simulink model "CarrotPlannerAlgorithm"  (R2022a)
settings: Solver=ode23s  StartTime=0.0  StopTime=inf  FixedStep=0.005  RelTol=1e-3
InitFcn:
  | RPInit
model workspace (MAT data in the model file):
  mapForSim : object (value not decoded)
  occGrid : robotics.BinaryOccupancyGrid (value not decoded)
undefined symbols (not defined in the file or in its folder): FloorSurface, Ref, RobotSurface, X, Y, Z
libraries: sm_lib x21, RoboticsPlayground x20, RP_Simulator_Components x15, nesl_utility x14
(part 2 of 2)

== stateflow chart CarrotPlannerAlgorithm/Vortex ==
  state TurningWest5
    LeftMotor=110;
    RightMotor=127;
  state TurningWest6
    LeftMotor=127;
    RightMotor=126;
  state TurningWest4
    LeftMotor=80;
    RightMotor=127;
  state TurningWest3
    LeftMotor=70;
    RightMotor=127;
  state rightFast8
    LeftMotor=125;
    RightMotor=127;
  state TurningWest
    LeftMotor=-40;
    RightMotor=80;
  state TurningWest2
    LeftMotor=40;
    RightMotor=127;
  state rightFast7
    LeftMotor=125;
    RightMotor=127;
  state StartingParameter
    LeftMotor=+127;
    RightMotor=+127;
  state TurningNorth
    LeftMotor=-40;
    RightMotor=80;
  state TurningNorth2
    LeftMotor=40;
    RightMotor=127;
  state TurningNorth3
    LeftMotor=70;
    RightMotor=127;
  state TurningNorth4
    LeftMotor=80;
    RightMotor=127;
  state TurningNorth5
    LeftMotor=110;
    RightMotor=127;
  state TurningNorth6
    LeftMotor=127;
    RightMotor=126;
  state TurningSouth6
    LeftMotor=126;
    RightMotor=127;
  state TurningSouth
    LeftMotor=-40;
    RightMotor=80;
  state TurningSouth2
    LeftMotor=40;
    RightMotor=127;
  state TurningSouth3
    LeftMotor=70;
    RightMotor=127;
  state TurningSouth4
    LeftMotor=80;
    RightMotor=127;
  state TurningSouth5
    LeftMotor=110;
    RightMotor=127;
  state rightFast10
    LeftMotor=127;
    RightMotor=125;
  state TurningSouth7
    LeftMotor=126;
    RightMotor=127;
  state TurningSouth11
    LeftMotor=80;
    RightMotor=-40;
  state TurningSouth12
    LeftMotor=127;
    RightMotor=40;
  state TurningSouth10
    LeftMotor=127;
    RightMotor=70;
  state TurningSouth9
    LeftMotor=127;
    RightMotor=80;
  state TurningSouth8
    LeftMotor=127;
    RightMotor=110;
  state rightFast9
    LeftMotor=127;
    RightMotor=125;
  state TurningSouth15
    LeftMotor=126;
    RightMotor=127;
  state TurningSouth16
    LeftMotor=-40;
    RightMotor=80;
  state TurningSouth17
    LeftMotor=40;
    RightMotor=127;
  state TurningSouth13
    LeftMotor=70;
    RightMotor=127;
  state TurningSouth18
    LeftMotor=80;
    RightMotor=127;
  state TurningSouth14
    LeftMotor=110;
    RightMotor=127;
  state TurningNorth9
    LeftMotor=-40;
    RightMotor=80;
  state TurningNorth12
    LeftMotor=40;
    RightMotor=127;
  state TurningNorth10
    LeftMotor=70;
    RightMotor=127;
  state TurningNorth11
    LeftMotor=80;
    RightMotor=127;
  state TurningNorth8
    LeftMotor=110;
    RightMotor=127;
  state TurningNorth7
    LeftMotor=126;
    RightMotor=127;
  state rightFast11
    LeftMotor=127;
    RightMotor=125;
  state TurningNorth15
    LeftMotor=0;
    RightMotor=0;
  rightFast7 -> StartingParameter [order 1] : [frontDist<0.3+(k*j)]{i=i+1;}
  rightFast8 -> StartingParameter [order 1] : [frontDist<0.3+(k*j)]{i=i+1;}
  rightFast8 -> TurningWest6 [order 2] : [180-angle>=0]
  TurningWest5 -> TurningWest6 : [180-angle>=0.1]
  TurningWest4 -> TurningWest5 : [180-angle<0.5]
  TurningWest3 -> TurningWest4 : [180-angle<2]
  StartingParameter -> TurningWest [order 2] : [frontDist<0.4+(k*j) && mod(i,3)==1 && rightDist<0.4+(k*j) && ~(j==4)]
  TurningWest2 -> TurningWest3 : [180-angle<5]
  TurningWest6 -> rightFast8 : [180-angle<0.1  || frontDist<0.3+(k*j)]
  TurningWest -> TurningWest2 : [180-angle<10]
  rightFast7 -> TurningNorth6 [order 2] : [180-angle<89.9]
  StartingParameter -> TurningNorth [order 1] : [frontDist<0.3+((k*j)-l*0.1) && mod(i,3)==0 && rightDist<0.3+(k*j) && ~(j==4)]
  TurningNorth -> TurningNorth2 : [180-angle<100]
  TurningNorth2 -> TurningNorth3 : [180-angle<95]
  TurningNorth3 -> TurningNorth4 : [180-angle<92]
  TurningNorth4 -> TurningNorth5 : [(180-angle<90.5)]
  TurningNorth5 -> TurningNorth6 : [180-angle<=(90.1)]
  (default) -> StartingParameter : {i=0, j=0,k=0.3,l=0}
  TurningNorth6 -> rightFast7 : [180-angle>=90 || frontDist<0.3+(k*j)]
  StartingParameter -> TurningNorth15 [order 3] : [j==4 && leftDist<0.1]
  rightFast11 -> StartingParameter [order 2] : [frontDist<0.3+(k*j)]{i=0;}
  TurningSouth6 -> StartingParameter : {i=i+1;}
  StartingParameter -> TurningSouth11 [order 4] : [mod(i,3)==0 && rightDist>=0.3+(k*j) && frontDist<4-(k*j) && ~(j==4)]
  StartingParameter -> TurningSouth [order 5] : [frontDist<0.3+((k*j)-l*0.1) && mod(i,3)==2 && rightDist<0.3+(k*j) && ~(j==4)]
  TurningSouth -> TurningSouth2 : [angle<100]
  TurningSouth2 -> TurningSouth3 : [angle<95]
  TurningSouth3 -> TurningSouth4 : [angle<92]
  TurningSouth4 -> TurningSouth5 : [angle<90.5]
  TurningSouth5 -> TurningSouth6 : [angle<=(90.1)]
  rightFast10 -> TurningSouth15 : [angle>90 || frontDist<0.3+(k*j)]
  TurningSouth15 -> rightFast10 [order 1] : [angle<=90.1 && ~(frontDist<0.3+(k*j))]
  TurningSouth11 -> TurningSouth12 : [180-angle<10]
  TurningSouth12 -> TurningSouth10 : [180-angle<5]
  TurningSouth10 -> TurningSouth9 : [180-angle<2]
  TurningSouth9 -> TurningSouth8 : [180-angle<0.5]
  TurningSouth8 -> TurningSouth7 : [180-angle<=0.1]
  TurningSouth7 -> rightFast9 : [180-angle>=0.1  || frontDist<0.3+(k*j)]
  rightFast9 -> TurningSouth7 [order 1] : [180-angle<0.1]
  rightFast9 -> TurningSouth16 [order 2] : [frontDist<0.3+(k*j) && rightDist<0.3+(k*j) && ~(j==4) ]{j=j+1;l=l+1}
  TurningSouth16 -> TurningSouth17 : [angle<100]
  TurningSouth17 -> TurningSouth13 : [angle<95]
  TurningSouth13 -> TurningSouth18 : [angle<92]
  TurningSouth18 -> TurningSouth14 : [angle<90.5]
  TurningSouth14 -> TurningSouth15 : [angle<=(90.1)]
  TurningNorth9 -> TurningNorth12 : [angle<10]
  TurningNorth12 -> TurningNorth10 : [angle<5]
  TurningNorth10 -> TurningNorth11 : [angle<2]
  TurningNorth11 -> TurningNorth8 : [(angle<0.5)]
  TurningNorth8 -> TurningNorth7 : [angle<=0.1]
  TurningSouth15 -> TurningNorth9 [order 2] : [frontDist<0.3+(k*j) && rightDist<0.3+(k*j)]
  TurningNorth7 -> rightFast11 : [angle>=0.1  || frontDist<0.3+(k*j)]
  rightFast11 -> TurningNorth7 [order 1] : [angle<0.1 && ~(frontDist<0.3+(k*j))]
  data: LeftMotor output; RightMotor output; frontDist input; leftDist input; rightDist input; angle input; i local; xpose input; ypose input; j local; k local; dir input; l local

== stateflow chart CarrotPlannerAlgorithm/S pattern1 ==
  state rightFast7
    LeftMotor=125;
    RightMotor=127;
  state ControlPart5
    LeftMotor=127;
    RightMotor=125;
  state rightFast6
    LeftMotor=127;
    RightMotor=126;
  state rightFast5
    LeftMotor=127;
    RightMotor=110;
  state leftFast5
    LeftMotor=110;
    RightMotor=127;
  state ControlPart6
    LeftMotor=126;
    RightMotor=127;
  state rightFast4
    LeftMotor=127;
    RightMotor=80;
  state leftFast4
    LeftMotor=80;
    RightMotor=127;
  state Initial1
    LeftMotor=127;
    RightMotor=+127;
  state rightFast1
    LeftMotor=80;
    RightMotor=-40;
  state rightFast2
    LeftMotor=127;
    RightMotor=40;
  state rightFast3
    LeftMotor=127;
    RightMotor=70;
  state leftFast1
    LeftMotor=-40;
    RightMotor=80;
  state leftFast3
    LeftMotor=70;
    RightMotor=127;
  state leftFast2
    LeftMotor=40;
    RightMotor=127;
  state Init1
    LeftMotor=-80;
    RightMotor=80;;
  state Init2
    LeftMotor=-50;
    RightMotor=50;
  state StartCond
    x = abs(xpose-xdesired);
    y = abs(ypose-ydesired);
    alfa = atan(y/x);
    alfa = rad2deg(alfa);
    alfa1=alfa;
    out=0;
  state Init3
    LeftMotor=-30;
    RightMotor=30;
  state Init7
    LeftMotor=123;
    RightMotor=120;
  state Init5
    LeftMotor=100;
    RightMotor=100;
  state Init6
    LeftMotor=120;
    RightMotor=121.3;
  state Init17
    out=0;
    LeftMotor=-80;
    RightMotor=80;
  state rightFast10
    LeftMotor=125;
    RightMotor=127;
  state abcd2
    LeftMotor=-50;
    RightMotor=50;
  state ControlPart8
    LeftMotor=127;
    RightMotor=125;
  state rightFast8
    LeftMotor=127;
    RightMotor=126;
  state rightFast11
    LeftMotor=127;
    RightMotor=110;
  state abcd
    LeftMotor=-30;
    RightMotor=30;
  state leftFast9
    LeftMotor=110;
    RightMotor=127;
  state ControlPart7
    LeftMotor=126;
    RightMotor=127;
  state abcd1
    LeftMotor=-10;
    RightMotor=10;
  state rightFast9
    LeftMotor=127;
    RightMotor=80;
  state leftFast10
    LeftMotor=80;
    RightMotor=127;
  state abcd3
    LeftMotor=3;
    RightMotor=-3;
  state Initial2
    LeftMotor=127;
    RightMotor=127;
  state rightFast14
    LeftMotor=80;
    RightMotor=-40;
  state rightFast12
    LeftMotor=127;
    RightMotor=40;
  state rightFast13
    LeftMotor=127;
    RightMotor=70;
  state leftFast6
    LeftMotor=-40;
    RightMotor=80;
  state leftFast7
    LeftMotor=70;
    RightMotor=127;
  state leftFast8
    LeftMotor=40;
    RightMotor=127;
  rightFast7 -> rightFast6 : [angle<0.1 || frontDist<0.3]
  rightFast6 -> rightFast7 [order 1] : [angle>=0.1 && ~(frontDist<0.3)]
  ControlPart5 -> ControlPart6 : [angle>179.9 || frontDist<0.3]
  ControlPart6 -> ControlPart5 [order 1] : [dir==0 &&angle>=0.1 && ~(frontDist<0.3)]
  rightFast6 -> Initial1 [order 2] : [(frontDist<0.3 &&mod(i,2)==0)]
  rightFast5 -> rightFast6 : [angle<(0.2)]{i=i+1;}
  rightFast4 -> rightFast5 : [angle>0&&angle<0.5]
  leftFast5 -> ControlPart6 : [180-angle<(0.2)]{i=i+1;}
  leftFast4 -> leftFast5 : [180-angle<0.5]
  ControlPart6 -> Initial1 [order 2] : [frontDist<0.3 &&mod(i,2)==1]
  (default) -> Initial1 : {i=0,j=0,k=0}
  rightFast3 -> rightFast4 : [angle>0&&angle<2]
  leftFast3 -> leftFast4 : [180-angle<2]
  Initial1 -> rightFast1 [order 1] : [frontDist<0.3 &&mod(i,2)==1 && ~(i==17)]
  Initial1 -> leftFast1 [order 3] : [frontDist<0.3 &&mod(i,2)==0 && ~(i==17)]
  rightFast1 -> rightFast2 : [angle>0&&angle<10]
  rightFast2 -> rightFast3 : [angle>0&&angle<5]
  leftFast1 -> leftFast2 : [180-angle<10]
  leftFast2 -> leftFast3 : [180-angle<5]
  Initial1 -> StartCond [order 2] : [i==17]{xdesired=4.8;ydesired=3;}
  StartCond -> Init1
  Init1 -> Init2 : [abs(angle-alfa)<3]
  Init2 -> Init3 : [abs(angle-alfa)<1]
  Init3 -> Init5 : [abs(angle-alfa)<0.2]
  Init5 -> Init7 [order 3] : [[angle-alfa<0.5]]
  Init6 -> Init5 [order 2] : [alfa-angle<0.005]
  Init7 -> Init5 [order 2] : [[[angle-alfa<0.1]]]
  Init5 -> Init6 [order 2] : [alfa-angle<0.1]
  Init7 -> Init17 [order 1] : [xdesired-xpose<0.005 && ydesired-ypose<0.005 ]
  Init5 -> Init17 [order 1] : [xdesired-xpose<0.005 && ydesired-ypose<0.005 ]
  Init6 -> Init17 [order 1] : [xdesired-xpose<0.005 && ydesired-ypose<0.005 ]
  Init17 -> abcd2 : [angle<10]
  rightFast10 -> rightFast8 : [angle<179.9 || frontDist<0.3]
  rightFast8 -> rightFast10 [order 1] : [angle>=180 && ~(frontDist<0.3)]
  abcd2 -> abcd : [angle<2]
  ControlPart8 -> ControlPart7 : [angle>0.1 || frontDist<0.3]
  ControlPart7 -> ControlPart8 [order 1] : [dir==0 &&angle<=0 && ~(frontDist<0.3)]
  rightFast8 -> Initial2 [order 2] : [(frontDist<0.3 &&mod(i,2)==0)]
  rightFast11 -> rightFast8 : [angle>179.8 && angle<180]{i=i+1;}
  abcd -> abcd1 : [angle<0.5]
  rightFast9 -> rightFast11 : [angle>179.5 && angle<180]
  leftFast9 -> ControlPart7 : [angle<(0.2)]{i=i+1;}
  leftFast10 -> leftFast9 : [angle<0.5]
  ControlPart7 -> Initial2 [order 2] : [frontDist<0.3 &&mod(i,2)==1]
  abcd1 -> abcd3 : [angle<0.2]
  rightFast13 -> rightFast9 : [angle>178 && angle<180]
  leftFast7 -> leftFast10 : [angle<2]
  abcd3 -> Initial2 : [0.1>angle]
  Initial2 -> rightFast14 [order 1] : [frontDist<0.3 &&mod(i,2)==1]
  Initial2 -> leftFast6 [order 2] : [frontDist<0.3 &&mod(i,2)==0]
  rightFast14 -> rightFast12 : [angle>170 && angle<180]
  rightFast12 -> rightFast13 : [angle>175 && angle<180]
  leftFast6 -> leftFast8 : [angle<10]
  leftFast8 -> leftFast7 : [angle<5]
  data: LeftMotor output; RightMotor output; frontDist input; leftDist input; rightDist input; angle input; i local; xpose input; ypose input; j local; k local; dir input; alfa1 output; out output; xdesired local; x local; ydesired local; y local; alfa local

== stateflow chart CarrotPlannerAlgorithm/Vortex3 ==
  state TurningWest5
    LeftMotor=110;
    RightMotor=127;
  state TurningWest6
    LeftMotor=127;
    RightMotor=126;
  state TurningWest4
    LeftMotor=80;
    RightMotor=127;
  state TurningWest3
    LeftMotor=70;
    RightMotor=127;
  state rightFast8
    LeftMotor=125;
    RightMotor=127;
  state TurningWest
    LeftMotor=-40;
    RightMotor=80;
  state TurningWest2
    LeftMotor=40;
    RightMotor=127;
  state rightFast7
    LeftMotor=125;
    RightMotor=127;
  state StartingParameter
    LeftMotor=+127;
    RightMotor=+127;
  state TurningNorth
    LeftMotor=-40;
    RightMotor=80;
  state TurningNorth2
    LeftMotor=40;
    RightMotor=127;
  state TurningNorth3
    LeftMotor=70;
    RightMotor=127;
  state TurningNorth4
    LeftMotor=80;
    RightMotor=127;
  state TurningNorth5
    LeftMotor=110;
    RightMotor=127;
  state TurningNorth6
    LeftMotor=127;
    RightMotor=126;
  state TurningSouth6
    LeftMotor=126;
    RightMotor=127;
  state TurningSouth
    LeftMotor=-40;
    RightMotor=80;
  state TurningSouth2
    LeftMotor=40;
    RightMotor=127;
  state TurningSouth3
    LeftMotor=70;
    RightMotor=127;
  state TurningSouth4
    LeftMotor=80;
    RightMotor=127;
  state TurningSouth5
    LeftMotor=110;
    RightMotor=127;
  state TurningSouth7
    LeftMotor=126;
    RightMotor=127;
  state TurningSouth11
    LeftMotor=80;
    RightMotor=-40;
  state TurningSouth12
    LeftMotor=127;
    RightMotor=40;
  state TurningSouth10
    LeftMotor=127;
    RightMotor=70;
  state TurningSouth9
    LeftMotor=127;
    RightMotor=80;
  state TurningSouth8
    LeftMotor=127;
    RightMotor=110;
  state StartCond
    x = abs(xpose-xdesired);
    y = abs(ypose-ydesired);
    alfa = atan(y/x);
    alfa = rad2deg(alfa);
    alfa1=alfa;
    out=0;
  state TurningWest15
    LeftMotor=127;
    RightMotor=126;
  state TurningWest7
    LeftMotor=127;
    RightMotor=126;
  state Init1
    LeftMotor=80;
    RightMotor=-80;;
  state Init2
    LeftMotor=50;
    RightMotor=-50;
  state TurningSouth23
    LeftMotor=-40;
    RightMotor=80;
  state TurningNorth23
    LeftMotor=126;
    RightMotor=127;
  state TurningNorth27
    LeftMotor=-40;
    RightMotor=80;
  state rightFast11
    LeftMotor=127;
    RightMotor=125;
  state TurningNorth18
    LeftMotor=-40;
    RightMotor=80;
  state rightFast9
    LeftMotor=127;
    RightMotor=125;
  state TurningNorth7
    LeftMotor=126;
    RightMotor=127;
  state TurningSouth16
    LeftMotor=-40;
    RightMotor=80;
  state Init4
    LeftMotor=10;
    RightMotor=-10;
  state Init3
    LeftMotor=30;
    RightMotor=-30;
  state TurningWest18
    LeftMotor=110;
    RightMotor=127;
  state TurningNorth20
    LeftMotor=110;
    RightMotor=127;
  state TurningNorth8
    LeftMotor=110;
    RightMotor=127;
  state TurningSouth17
    LeftMotor=40;
    RightMotor=127;
  state TurningWest9
    LeftMotor=110;
    RightMotor=127;
  state TurningSouth24
    LeftMotor=40;
    RightMotor=127;
  state TurningNorth29
    LeftMotor=40;
    RightMotor=127;
  state TurningNorth16
    LeftMotor=40;
    RightMotor=127;
  state TurningSouth13
    LeftMotor=70;
    RightMotor=127;
  state TurningNorth11
    LeftMotor=80;
    RightMotor=127;
  state Init7
    LeftMotor=120;
    RightMotor=123;
  state Init5
    LeftMotor=100;
    RightMotor=100;
  state Init6
    LeftMotor=121.3;
    RightMotor=120;
  state TurningNorth28
    LeftMotor=70;
    RightMotor=127;
  state TurningNorth14
    LeftMotor=70;
    RightMotor=127;
  state TurningSouth21
    LeftMotor=70;
    RightMotor=127;
  state TurningNorth19
    LeftMotor=80;
    RightMotor=127;
  state TurningWest13
    LeftMotor=80;
    RightMotor=127;
  state TurningWest11
    LeftMotor=80;
    RightMotor=127;
  state TurningSouth18
    LeftMotor=80;
    RightMotor=127;
  state TurningNorth10
    LeftMotor=70;
    RightMotor=127;
  state TurningWest16
    LeftMotor=70;
    RightMotor=127;
  state TurningNorth25
    LeftMotor=80;
    RightMotor=127;
  state TurningWest10
    LeftMotor=70;
    RightMotor=127;
  state TurningSouth19
    LeftMotor=80;
    RightMotor=127;
  state TurningNorth13
    LeftMotor=80;
    RightMotor=127;
  state TurningNorth21
    LeftMotor=70;
    RightMotor=127;
  state Init17
    out=0;
    LeftMotor=80;
    RightMotor=-80;
  state TurningSouth14
    LeftMotor=110;
    RightMotor=127;
  state TurningNorth12
    LeftMotor=40;
    RightMotor=127;
  state TurningWest17
    LeftMotor=40;
    RightMotor=127;
  state TurningNorth30
    LeftMotor=110;
    RightMotor=127;
  state TurningWest12
    LeftMotor=40;
    RightMotor=127;
  state TurningNorth15
    LeftMotor=110;
    RightMotor=127;
  state TurningSouth20
    LeftMotor=110;
    RightMotor=127;
  state TurningNorth22
    LeftMotor=40;
    RightMotor=127;
  state abcd2
    LeftMotor=50;
    RightMotor=-50;
  state TurningSouth15
    LeftMotor=126;
    RightMotor=127;
  state rightFast10
    LeftMotor=127;
    RightMotor=125;
  state TurningNorth9
    LeftMotor=-40;
    RightMotor=80;
  state TurningWest14
    LeftMotor=-40;
    RightMotor=80;
  state TurningNorth26
    LeftMotor=127;
    RightMotor=126;
  state TurningWest8
    LeftMotor=-40;
    RightMotor=80;
  state TurningSouth22
    LeftMotor=126;
    RightMotor=127;
  state TurningNorth17
    LeftMotor=127;
    RightMotor=126;
  state TurningNorth24
    LeftMotor=-40;
    RightMotor=80;
  state abcd
    LeftMotor=30;
    RightMotor=-30;
  state abcd1
    LeftMotor=10;
    RightMotor=-10;
  state abcd3
    LeftMotor=3;
    RightMotor=-3;
  state Duz
    LeftMotor=126;
    RightMotor=127;
  state TurningWest21
    LeftMotor=127;
    RightMotor=126;
  state TurningSouth25
    LeftMotor=-40;
    RightMotor=80;
  state TurningNorth40
    LeftMotor=126;
    RightMotor=127;
  state TurningNorth33
    LeftMotor=-40;
    RightMotor=80;
  state TurningWest24
    LeftMotor=110;
    RightMotor=127;
  state TurningSouth28
    LeftMotor=40;
    RightMotor=127;
  state TurningNorth42
    LeftMotor=110;
    RightMotor=127;
  state TurningNorth35
    LeftMotor=40;
    RightMotor=127;
  state TurningSouth27
    LeftMotor=70;
    RightMotor=127;
  state TurningNorth38
    LeftMotor=80;
    RightMotor=127;
  state TurningWest19
    LeftMotor=80;
    RightMotor=127;
  state TurningNorth34
    LeftMotor=70;
    RightMotor=127;
  state TurningWest22
    LeftMotor=70;
    RightMotor=127;
  state TurningSouth29
    LeftMotor=80;
    RightMotor=127;
  state TurningNorth31
    LeftMotor=80;
    RightMotor=127;
  state TurningNorth41
    LeftMotor=70;
    RightMotor=127;
  state TurningWest23
    LeftMotor=40;
    RightMotor=127;
  state TurningNorth36
    LeftMotor=110;
    RightMotor=127;
  state TurningSouth30
    LeftMotor=110;
    RightMotor=127;
  state TurningNorth39
    LeftMotor=40;
    RightMotor=127;
  state TurningWest20
    LeftMotor=-40;
    RightMotor=80;
  state TurningSouth26
    LeftMotor=126;
    RightMotor=127;
  state TurningNorth32
    LeftMotor=127;
    RightMotor=126;
  state TurningNorth37
    LeftMotor=-40;
    RightMotor=80;
  rightFast7 -> StartingParameter [order 1] : [frontDist<0.3+(k*j)]{i=i+1;}
  rightFast8 -> StartingParameter [order 1] : [frontDist<0.3+(k*j)]{i=i+1;}
  rightFast8 -> TurningWest6 [order 2] : [180-angle>=0]
  TurningWest5 -> TurningWest6 : [180-angle>=0.1]
  TurningWest4 -> TurningWest5 : [180-angle<0.5]
  TurningWest3 -> TurningWest4 : [180-angle<2]
  StartingParameter -> TurningWest [order 2] : [frontDist<0.3+(k*j) && mod(i,3)==1 && rightDist<0.3+(k*j) || leftDist<0.3]
  TurningWest2 -> TurningWest3 : [180-angle<5]
  TurningWest6 -> rightFast8 : [180-angle<0.1  || frontDist<0.3+(k*j)]
  TurningWest -> TurningWest2 : [180-angle<10]
  rightFast7 -> TurningNorth6 [order 2] : [180-angle<89.9]
  StartingParameter -> TurningNorth [order 1] : [frontDist<0.2+((k*j)) && mod(i,3)==0 && rightDist<0.3+(k*j)  || leftDist<0.3]
  TurningNorth -> TurningNorth2 : [180-angle<100]
  TurningNorth2 -> TurningNorth3 : [180-angle<95]
  TurningNorth3 -> TurningNorth4 : [180-angle<92]
  TurningNorth4 -> TurningNorth5 : [(180-angle<90.5)]
  TurningNorth5 -> TurningNorth6 : [180-angle<=(90.1)]
  (default) -> StartingParameter : {i=0, j=0,k=0.3,l=0}
  TurningNorth6 -> rightFast7 : [180-angle>=90 || frontDist<0.3+(k*j)]
  rightFast11 -> StartingParameter [order 3] : [frontDist<0.3+(k*j)]{i=0;}
  TurningSouth6 -> StartingParameter : {i=i+1;}
  StartingParameter -> TurningSouth11 [order 3] : [mod(i,3)==0 && rightDist>=0.3+(k*j) && frontDist<4-(k*j)  || leftDist<0.3]
  StartingParameter -> TurningSouth [order 4] : [frontDist<0.3+((k*j)) && mod(i,3)==2 && rightDist<0.3+(k*j)  || leftDist<0.3]
  TurningSouth -> TurningSouth2 : [angle<100]
  TurningSouth2 -> TurningSouth3 : [angle<95]
  TurningSouth3 -> TurningSouth4 : [angle<92]
  TurningSouth4 -> TurningSouth5 : [angle<90.5]
  TurningSouth5 -> TurningSouth6 : [angle<=(90.1)]
  TurningSouth11 -> TurningSouth12 : [180-angle<10]
  TurningSouth12 -> TurningSouth10 : [180-angle<5]
  TurningSouth10 -> TurningSouth9 : [180-angle<2]
  TurningSouth9 -> TurningSouth8 : [180-angle<0.5]
  TurningSouth8 -> TurningSouth7 : [180-angle<=0.1]
  TurningSouth7 -> rightFast9 : [180-angle>=0.1  || frontDist<0.3+(k*j)]
  rightFast9 -> TurningSouth7 [order 1] : [180-angle<0.1]
  TurningWest15 -> StartCond : [frontDist<=1.7]{xdesired=3;ydesired=3.6;}
  StartCond -> Init1
  Init1 -> Init2 : [abs(angle-alfa)<5]
  TurningWest7 -> TurningSouth23 : [frontDist<1.5]
  TurningNorth23 -> TurningNorth27 : [frontDist<0.8]
  rightFast11 -> TurningNorth18 [order 2] : [frontDist<=3 && l==8]
  rightFast11 -> TurningNorth7 [order 1] : [angle<0.1 && ~(frontDist<0.3+(k*j))]
  rightFast9 -> TurningSouth16 [order 2] : [frontDist<0.3+(k*j) && rightDist<0.3+(k*j) || leftDist<0.3]{j=j+1;l=l+1}
  Init2 -> Init3 : [abs(angle-alfa)<3]
  TurningSouth23 -> TurningSouth24 : [angle<100]
  TurningNorth20 -> TurningNorth23 : [angle<=0.1]
  TurningNorth27 -> TurningNorth29 : [180-angle<100]
  TurningWest18 -> TurningWest15 : [180-angle>=0.1]
  TurningNorth7 -> rightFast11 : [angle>=0.1  || frontDist<0.3+(k*j)]
  TurningWest9 -> TurningWest7 : [180-angle>=0.1]
  TurningNorth18 -> TurningNorth16 : [180-angle<100]
  TurningNorth8 -> TurningNorth7 : [angle<=0.1]
  TurningSouth16 -> TurningSouth17 : [angle<100]
  Init3 -> Init4 : [abs(angle-alfa)<1]
  Init4 -> Init5 : [abs(angle-alfa)<0.3]
  TurningNorth19 -> TurningNorth20 : [(angle<0.5)]
  TurningNorth11 -> TurningNorth8 : [(angle<0.5)]
  TurningSouth17 -> TurningSouth13 : [angle<95]
  TurningSouth24 -> TurningSouth21 : [angle<95]
  TurningNorth29 -> TurningNorth28 : [180-angle<95]
  TurningWest13 -> TurningWest18 : [180-angle<0.5]
  TurningNorth16 -> TurningNorth14 : [180-angle<95]
  TurningWest11 -> TurningWest9 : [180-angle<0.5]
  Init5 -> Init7 [order 3] : [angle-alfa<0.5]
  Init6 -> Init5 [order 2] : [alfa-angle<0.005]
  Init7 -> Init5 [order 2] : [angle-alfa<0.1]
  Init5 -> Init6 [order 2] : [alfa-angle<0.1]
  TurningSouth13 -> TurningSouth18 : [angle<92]
  TurningNorth10 -> TurningNorth11 : [angle<2]
  Init7 -> Init17 [order 1] : [xdesired-xpose<0.005 && ydesired-ypose<0.005 ]
  Init6 -> Init17 [order 1] : [xdesired-xpose<0.005 && ydesired-ypose<0.005 ]
  Init5 -> Init17 [order 1] : [xdesired-xpose<0.005 && ydesired-ypose<0.005 ]
  TurningNorth28 -> TurningNorth25 : [180-angle<92]
  TurningNorth14 -> TurningNorth13 : [180-angle<92]
  TurningSouth21 -> TurningSouth19 : [angle<92]
  TurningNorth21 -> TurningNorth19 : [angle<2]
  TurningWest16 -> TurningWest13 : [180-angle<2]
  TurningWest10 -> TurningWest11 : [180-angle<2]
  TurningSouth18 -> TurningSouth14 : [angle<90.5]
  TurningNorth12 -> TurningNorth10 : [angle<5]
  TurningNorth25 -> TurningNorth30 : [(180-angle<90.5)]
  TurningWest17 -> TurningWest16 : [180-angle<5]
  TurningSouth19 -> TurningSouth20 : [angle<90.5]
  TurningNorth13 -> TurningNorth15 : [(180-angle<90.5)]
  TurningNorth22 -> TurningNorth21 : [angle<5]
  TurningWest12 -> TurningWest10 : [180-angle<5]
  Init17 -> abcd2 : [angle<10]
  TurningSouth14 -> TurningSouth15 : [angle<=(90.1)]{l=l+1;}
  TurningNorth9 -> TurningNorth12 : [angle<10]
  TurningNorth30 -> TurningNorth26 : [180-angle<=(90.1)]
  TurningWest14 -> TurningWest17 : [180-angle<10]
  TurningNorth15 -> TurningNorth17 : [180-angle<=(90.1)]
  TurningSouth20 -> TurningSouth22 : [angle<=(90.1)]
  TurningNorth24 -> TurningNorth22 : [angle<10]
  TurningWest8 -> TurningWest12 : [180-angle<10]
  TurningSouth15 -> rightFast10 [order 1] : [angle<=90.1 && ~(frontDist<0.3+(k*j))]
  abcd2 -> abcd : [angle<2]
  TurningSouth15 -> TurningNorth9 [order 2] : [frontDist<0.3+(k*j) && rightDist<0.3+(k*j)  || leftDist<0.3]
  rightFast10 -> TurningSouth15 : [angle>90 || frontDist<0.3+(k*j)]
  TurningNorth26 -> TurningWest14 : [frontDist<=3.6]
  TurningSouth22 -> TurningNorth24 : [frontDist<1.8]
  TurningNorth17 -> TurningWest8 : [frontDist<=3.2]
  abcd -> abcd1 : [angle<0.5]
  abcd1 -> abcd3 : [angle<0.2]
  abcd3 -> Duz : [0.1>=angle]
  Duz -> TurningNorth33 : [frontDist<=1.5]
  TurningWest21 -> TurningSouth25 : [frontDist<2.2]
  TurningSouth25 -> TurningNorth37 [order 2] : [frontDist<1.4]
  TurningSouth25 -> TurningSouth28 [order 1] : [angle<100]
  TurningNorth42 -> TurningNorth40 : [angle<=0.1]
  TurningWest24 -> TurningWest21 : [180-angle>=0.1]
  TurningNorth33 -> TurningNorth35 : [180-angle<100]
  TurningSouth28 -> TurningSouth27 : [angle<95]
  TurningNorth38 -> TurningNorth42 : [(angle<0.5)]
  TurningWest19 -> TurningWest24 : [180-angle<0.5]
  TurningNorth35 -> TurningNorth34 : [180-angle<95]
  TurningSouth27 -> TurningSouth29 : [angle<92]
  TurningNorth41 -> TurningNorth38 : [angle<2]
  TurningWest22 -> TurningWest19 : [180-angle<2]
  TurningNorth34 -> TurningNorth31 : [180-angle<92]
  TurningSouth29 -> TurningSouth30 : [angle<90.5]
  TurningNorth31 -> TurningNorth36 : [(180-angle<90.5)]
  TurningWest23 -> TurningWest22 : [180-angle<5]
  TurningNorth39 -> TurningNorth41 : [angle<5]
  TurningNorth36 -> TurningNorth32 : [180-angle<=(90.1)]
  TurningSouth30 -> TurningSouth26 : [angle<=(90.1)]
  TurningWest20 -> TurningWest23 : [180-angle<10]
  TurningNorth37 -> TurningNorth39 : [angle<10]
  TurningNorth32 -> TurningWest20 : [frontDist<1.4]
  data: LeftMotor output; RightMotor output; frontDist input; leftDist input; rightDist input; angle input; i local; xpose input; ypose input; j local; k local; dir input; l local; xdesired local; y local; alfa local; ydesired local; x local; alfa1 output; out output

== matlab function CarrotPlannerAlgorithm/MATLAB Function ==
  data: u input; y output
function y = fcn(u)
    if u<0
        y=0;
    else
        y=1;
    end

end

== stateflow chart CarrotPlannerAlgorithm/S pattern ==
  note: frontdistance'yi buraya ekleyip dene
  state rightFast7
    LeftMotor=125;
    RightMotor=127;
  state ControlPart5
    LeftMotor=127;
    RightMotor=125;
  state rightFast6
    LeftMotor=127;
    RightMotor=126;
  state rightFast5
    LeftMotor=127;
    RightMotor=110;
  state leftFast5
    LeftMotor=110;
    RightMotor=127;
  state ControlPart6
    LeftMotor=126;
    RightMotor=127;
  state rightFast4
    LeftMotor=127;
    RightMotor=80;
  state leftFast4
    LeftMotor=80;
    RightMotor=127;
  state Initial1
    LeftMotor=127;
    RightMotor=+127;
  state rightFast1
    LeftMotor=80;
    RightMotor=-40;
  state rightFast2
    LeftMotor=127;
    RightMotor=40;
  state rightFast3
    LeftMotor=127;
    RightMotor=70;
  state leftFast1
    LeftMotor=-40;
    RightMotor=80;
  state leftFast3
    LeftMotor=70;
    RightMotor=127;
  state leftFast2
    LeftMotor=40;
    RightMotor=127;
  state Stop
    LeftMotor=127;
    RightMotor=127;
  rightFast7 -> rightFast6 : [angle<0.1 || frontDist<0.3]
  rightFast6 -> rightFast7 [order 1] : [angle>=0.1 && ~(frontDist<0.3)]
  ControlPart5 -> ControlPart6 : [angle>179.9 || frontDist<0.3]
  ControlPart6 -> ControlPart5 [order 1] : [dir==0 && angle>=0.1 && ~(frontDist<0.3)]
  rightFast6 -> Initial1 [order 2] : [[frontDist<0.3 &&mod(i,2)==0]]
  rightFast5 -> rightFast6 : [angle<(0.2)]{i=i+1;}
  rightFast4 -> rightFast5 : [angle>0&&angle<0.5]
  leftFast5 -> ControlPart6 : [180-angle<(0.2)]{i=i+1;}
  leftFast4 -> leftFast5 : [180-angle<0.5]
  ControlPart6 -> Initial1 [order 2] : [frontDist<0.3 &&mod(i,2)==1]
  (default) -> Initial1 : {i=0,j=0,k=0}
  rightFast3 -> rightFast4 : [angle>0&&angle<2]
  leftFast3 -> leftFast4 : [180-angle<2]
  Initial1 -> rightFast1 [order 1] : [frontDist<0.3 &&mod(i,2)==1]
  Initial1 -> leftFast1 [order 3] : [frontDist<0.3 &&mod(i,2)==0]
  rightFast1 -> rightFast2 : [angle>0&&angle<10]
  rightFast2 -> rightFast3 : [angle>0&&angle<5]
  leftFast1 -> leftFast2 : [180-angle<10]
  leftFast2 -> leftFast3 : [180-angle<5]
  Initial1 -> Stop [order 2] : [i==18 && frontDist<0.3]
  data: LeftMotor output; RightMotor output; frontDist input; leftDist input; rightDist input; angle input; i local; xpose input; ypose input; j local; k local; dir input
